simulink subsystem "Guiado2"  (R2021b)
settings: Solver=VariableStepAuto  StartTime=0.0  StopTime=10.0  RelTol=1e-3
values from neighbouring files (symbols this model uses):
  fp = [t1;t2;t3]    [creacionestructurasborrador.m]    (also in flight_plan.m = [sid,wps,iap]; flight_plan_eval.m = [t1;tabla2;t3]; flight_plan_old.m = [sid,wps,iap]; flight_plan_struct.m = [t1;tabla2;t3])
libraries: simulink x5
settings Model: Creator=patri  LastModifiedBy=verti

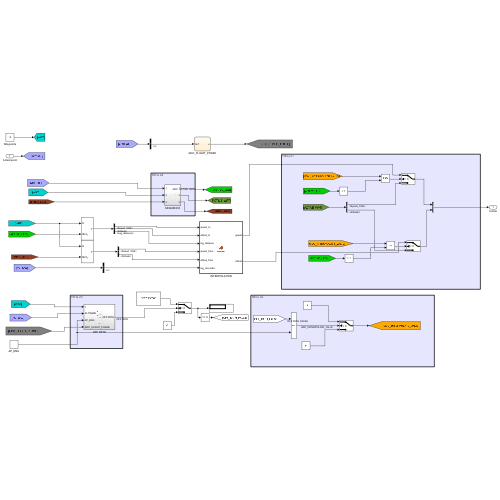
[thumbnail: Simulink's stored preview of the top-level diagram]
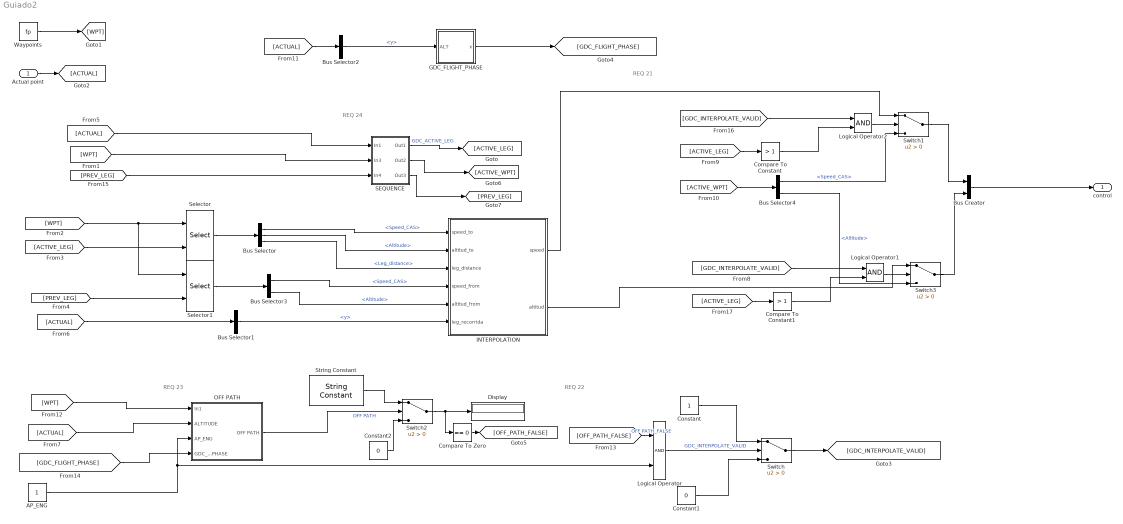
== system Guiado2 ==
  note: REQ 24
  note: REQ 23
  note: REQ 22
  note: REQ 21
  Actual point : Inport  RequirementInfo={} %GIDa_16dc30b3_4c57_4f20_ae6f_49b6e7f70ca9
  AP_ENG : Constant  RequirementInfo={} %GIDa_6cfd0b15_e0b7_412e_b898_13df53d186b9
  Bus Creator : BusCreator  RequirementInfo={} %GIDa_f95eb603_7edc_47e9_9511_efe566d1f221  Inputs=2
  Bus Selector : BusSelector  RequirementInfo={} %GIDa_748c13b4_26a4_4f06_b41f_6c0f351aa6e1  OutputSignals=Speed_CAS,Altitude,Leg_distance
  Bus Selector1 : BusSelector  RequirementInfo={} %GIDa_3209a6ab_bd8c_441c_92f5_266385c658f5  OutputSignals=x; y; z; phi; theta; psi.y
  Bus Selector2 : BusSelector  RequirementInfo={} %GIDa_66241123_1541_4933_9326_b685100fe374  OutputSignals=x; y; z; phi; theta; psi.y
  Bus Selector3 : BusSelector  RequirementInfo={} %GIDa_962e6f27_d2e9_4d95_8ffb_528ca1f04bd7  OutputSignals=Speed_CAS,Altitude
  Bus Selector4 : BusSelector  RequirementInfo={} %GIDa_8319d33c_1374_4958_9d6f_b54157dc937b  OutputSignals=Speed_CAS,Altitude
  Compare To Constant : simulink/Logic and Bit Operations/Compare To Constant  relop=>  const=1  OutDataTypeStr=boolean
  Compare To Constant1 : simulink/Logic and Bit Operations/Compare To Constant  relop=>  const=1  OutDataTypeStr=boolean
  Compare To Zero : simulink/Logic and Bit Operations/Compare To Zero  relop===  OutDataTypeStr=boolean
  Constant : Constant  RequirementInfo={} %GIDa_b37b12f2_4207_4d8d_8f51_6f8b678f3f25
  Constant1 : Constant  RequirementInfo={} %GIDa_9998b814_7f70_4580_aaca_dde72b20b372  Value=0
  Constant2 : Constant  RequirementInfo={} %GIDa_22a48ef9_4669_4f4b_8c84_0df911214b19  Value=0
  Display : Display
      settings: RequirementInfo={} %GIDa_b98bbcc7_d7c3_4a86_b2f1_97de43cdc8ad
  GDC_FLIGHT_PHASE : Stateflow chart  RequirementInfo={} %GIDa_6ca26d66_91a8_4b10_b43c_38c0903f28df  TreatAsAtomicUnit=on
  INTERPOLATION : MATLAB Function  RequirementInfo={} %GIDa_00da5b89_cd18_4ad3_bdd9_46f4b2278232  TreatAsAtomicUnit=on
  Logical Operator : Logic  RequirementInfo={} %GIDa_b237b72d_01a0_4ce8_b8fa_48e4c02eadaf  AllPortsSameDT=off  OutDataTypeStr=boolean
  Logical Operator1 : Logic  RequirementInfo={} %GIDa_3d17652f_edbe_41ba_a049_3408f2c4d262  AllPortsSameDT=off  OutDataTypeStr=boolean
  Logical Operator2 : Logic  RequirementInfo={} %GIDa_1178bee0_2321_439a_8aef_ffe83aa0f831  AllPortsSameDT=off  OutDataTypeStr=boolean
  OFF PATH : Subsystem  RequirementInfo={} %GIDa_e64eeec9_5eff_4758_836b_1b8b16284f0e
  SEQUENCE : Subsystem  RequirementInfo={} %GIDa_19bbec03_9c6d_4828_8024_6321fbffa4bc
  Selector : Selector  RequirementInfo={} %GIDa_52603b66_c8a4_4acb_b10d_5686338dd3d7  InputPortWidth=12  IndexOptions=Index vector (port)  Indices=[1 3]  OutputSizes=1
  Selector1 : Selector  RequirementInfo={} %GIDa_aadcde5b_c971_450e_aee0_b769e6a2f6d5  InputPortWidth=12  IndexOptions=Index vector (port)  Indices=[1 3]  OutputSizes=1
  String Constant : StringConstant  RequirementInfo={} %GIDa_0fff4776_2fb3_4bfd_9582_badec0246361  String="\"OFF PATH\""
  Switch : Switch  RequirementInfo={} %GIDa_7dce933e_33fe_4e3b_ae91_f92ffa975dd8  Criteria=u2 > Threshold
  Switch1 : Switch  RequirementInfo={} %GIDa_97a5f68e_f779_45d0_8fdd_ea3c790676b8  Criteria=u2 > Threshold
  Switch2 : Switch  RequirementInfo={} %GIDa_40c3c411_b3ce_405b_a9d1_145fd5b4c1df  Criteria=u2 > Threshold
  Switch3 : Switch  RequirementInfo={} %GIDa_aa545fae_3300_4656_9f8b_8d88f1b9a628  Criteria=u2 > Threshold
  Waypoints : Constant  RequirementInfo={} %GIDa_99d4dde1_a944_4af8_abed_c7d03318dd1c  Value=fp  OutDataTypeStr=Bus: BUS_FP
  control : Outport  RequirementInfo={} %GIDa_f06892af_3b8f_4cad_820d_58187372560f
  wires:
  SEQUENCE/1(Out1) -> [ACTIVE_LEG]  "GDC_ACTIVE_LEG"
  [PREV_LEG] -> SEQUENCE/3(In4)
  Waypoints/1 -> [WPT]
  [WPT] -> SEQUENCE/2(In3)
  [WPT] -> Selector/1, Selector1/1
  Selector/1 -> Bus Selector/1
  [ACTIVE_LEG] -> Selector/2
  Bus Selector/1 -> INTERPOLATION/1(speed_to)  "<Speed_CAS>"
  Bus Selector/2 -> INTERPOLATION/2(altitud_to)  "<Altitude>"
  Actual point/1 -> [ACTUAL]
  [ACTUAL] -> SEQUENCE/1(In1)
  [ACTUAL] -> Bus Selector1/1
  [ACTUAL] -> OFF PATH/2(ALTITUDE)
  AP_ENG/1 -> Logical Operator/2, OFF PATH/3(AP_ENG)
  OFF PATH/1(OFF PATH) -> Switch2/2  "OFF PATH"
  Logical Operator/1 -> Switch/2  "GDC_INTERPOLATE_VALID"
  Switch/1 -> [GDC_INTERPOLATE_VALID]
  Constant/1 -> Switch/1
  Constant1/1 -> Switch/3
  [GDC_INTERPOLATE_VALID] -> Logical Operator2/1
  [ACTIVE_LEG] -> Compare To Constant/1
  Compare To Constant/1 -> Logical Operator2/2
  Logical Operator2/1 -> Switch1/2
  Bus Selector2/1 -> GDC_FLIGHT_PHASE/1(ALT)  "<y>"
  [ACTUAL] -> Bus Selector2/1
  GDC_FLIGHT_PHASE/1(x) -> [GDC_FLIGHT_PHASE]
  [WPT] -> OFF PATH/1(In1)
  String Constant/1 -> Switch2/1
  Switch2/1 -> Compare To Zero/1, Display/1
  Constant2/1 -> Switch2/3
  [OFF_PATH_FALSE] -> Logical Operator/1  "OFF PATH_FALSE"
  SEQUENCE/2(Out2) -> [ACTIVE_WPT]
  SEQUENCE/3(Out3) -> [PREV_LEG]
  [GDC_FLIGHT_PHASE] -> OFF PATH/4(GDC_FLIGHT_PHASE)
  [PREV_LEG] -> Selector1/2
  Selector1/1 -> Bus Selector3/1
  Bus Selector3/1 -> INTERPOLATION/4(speed_from)  "<Speed_CAS>"
  Bus Selector3/2 -> INTERPOLATION/5(altitud_from)  "<Altitude>"
  INTERPOLATION/1(speed) -> Switch1/1
  [ACTIVE_WPT] -> Bus Selector4/1
  Bus Selector4/1 -> Switch1/3  "<Speed_CAS>"
  INTERPOLATION/2(altitud) -> Switch3/1
  Compare To Constant1/1 -> Logical Operator1/2
  [ACTIVE_LEG] -> Compare To Constant1/1
  [GDC_INTERPOLATE_VALID] -> Logical Operator1/1
  Logical Operator1/1 -> Switch3/2
  Bus Selector4/2 -> Switch3/3  "<Altitude>"
  Bus Creator/1 -> control/1
  Switch1/1 -> Bus Creator/1
  Switch3/1 -> Bus Creator/2
  Bus Selector/3 -> INTERPOLATION/3(leg_distance)  "<Leg_distance>"
  Bus Selector1/1 -> INTERPOLATION/6(leg_recorrida)  "<y>"
  Compare To Zero/1 -> [OFF_PATH_FALSE]

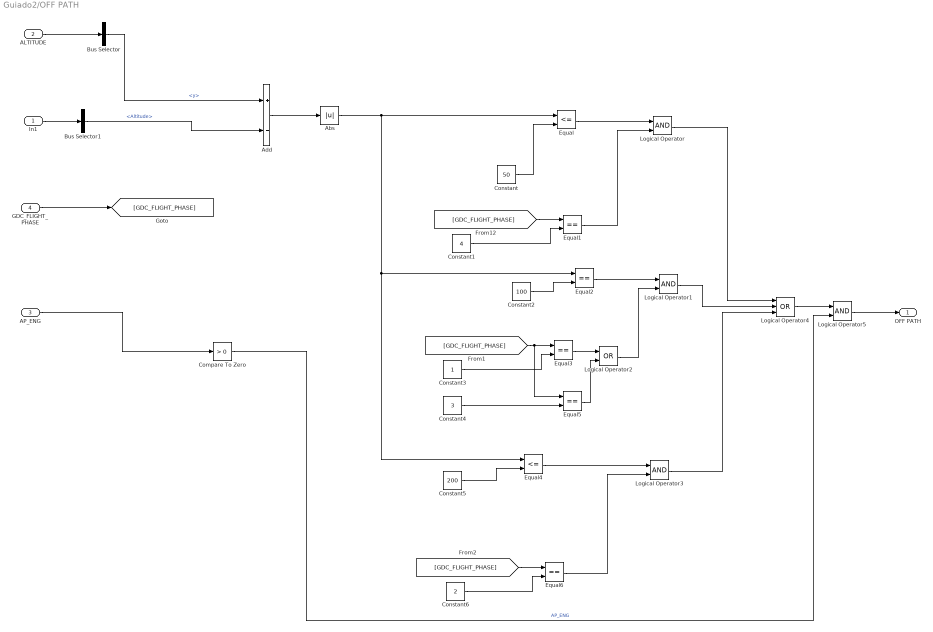
== system Guiado2/OFF PATH ==
  In1 : Inport  RequirementInfo={} %GIDa_62d6845d_2c83_4218_8ed5_ea4377ab5151
  ALTITUDE : Inport  RequirementInfo={} %GIDa_9ea31f00_8010_42f0_928c_ddcfbd884370  Port=2
  AP_ENG : Inport  RequirementInfo={} %GIDa_ee91ff1a_ab3d_4807_8f89_07a74f131ae5  Port=3
  GDC_FLIGHT_PHASE : Inport  RequirementInfo={} %GIDa_dae7e5fb_86bd_4482_b14f_0edc6d3d11c9  Port=4
  Abs : Abs  RequirementInfo={} %GIDa_3a6c06fc_ca93_4cf4_922a_74b5cd0bf12b
  Add : Sum  RequirementInfo={} %GIDa_62393710_84da_4880_81fd_b48a5142b0ab  Inputs=+-
  Bus Selector : BusSelector  RequirementInfo={} %GIDa_3537ae3d_a00e_41d7_b122_9f4ee9b7e234  OutputSignals=x; y; z; phi; theta; psi.y
  Bus Selector1 : BusSelector  RequirementInfo={} %GIDa_83aecc4c_d4cc_4dc5_b0bf_080722190f3a  OutputSignals=Altitude
  Compare To Zero : simulink/Logic and Bit Operations/Compare To Zero  RequirementInfo={} %GIDa_10f91483_6a15_433b_9377_e6e7499d1f49  relop=>  OutDataTypeStr=boolean
  Constant : Constant  RequirementInfo={} %GIDa_9b56d611_43a9_4f81_8a37_8310ab01972c  Value=50
  Constant1 : Constant  RequirementInfo={} %GIDa_6c81b280_bb28_483b_9de7_a5d2e6c184b3  Value=4
  Constant2 : Constant  RequirementInfo={} %GIDa_43ae1b03_ffdd_4284_a340_920d10f39b4e  Value=100
  Constant3 : Constant  RequirementInfo={} %GIDa_2899eea0_8d79_4841_acad_6c949baede0c
  Constant4 : Constant  RequirementInfo={} %GIDa_023f6fee_60f9_4c0a_9384_cd2105696549  Value=3
  Constant5 : Constant  RequirementInfo={} %GIDa_bf05bd0f_ad96_4653_ba6c_864afd652a73  Value=200
  Constant6 : Constant  RequirementInfo={} %GIDa_fbc4b4dc_b940_4f18_bcc6_343711a58847  Value=2
  Equal : RelationalOperator  RequirementInfo={} %GIDa_41fc17ac_0583_4b32_a798_806287f1de59  Operator=<=  OutDataTypeStr=boolean  RndMeth=Simplest
  Equal1 : RelationalOperator  RequirementInfo={} %GIDa_6b358ab3_1c30_4203_b31d_1b7c47e65652  Operator===  OutDataTypeStr=boolean  RndMeth=Simplest
  Equal2 : RelationalOperator  RequirementInfo={} %GIDa_a1929ec3_10c6_4581_ba38_0b3e6f4a191d  Operator===  OutDataTypeStr=boolean  RndMeth=Simplest
  Equal3 : RelationalOperator  RequirementInfo={} %GIDa_ee58c8fd_0997_4c1b_9fda_8de655ddb8c2  Operator===  OutDataTypeStr=boolean  RndMeth=Simplest
  Equal4 : RelationalOperator  RequirementInfo={} %GIDa_40b0daee_de42_4601_9a17_7606db32d086  Operator=<=  OutDataTypeStr=boolean  RndMeth=Simplest
  Equal5 : RelationalOperator  RequirementInfo={} %GIDa_144482dd_7c5e_44de_80d4_0aae76d53f67  Operator===  OutDataTypeStr=boolean  RndMeth=Simplest
  Equal6 : RelationalOperator  RequirementInfo={} %GIDa_2cde3331_25b0_452d_90eb_a86eb0afbb20  Operator===  OutDataTypeStr=boolean  RndMeth=Simplest
  Logical Operator : Logic  RequirementInfo={} %GIDa_948a8364_549f_4376_beca_c4b6c0c4cff5  AllPortsSameDT=off  OutDataTypeStr=boolean
  Logical Operator1 : Logic  RequirementInfo={} %GIDa_cdaccc45_64a9_4082_a1c5_823a8b02242a  AllPortsSameDT=off  OutDataTypeStr=boolean
  Logical Operator2 : Logic  RequirementInfo={} %GIDa_a0c82861_09a2_4c7b_9dd2_c1b7ada60be2  Operator=OR  AllPortsSameDT=off  OutDataTypeStr=boolean
  Logical Operator3 : Logic  RequirementInfo={} %GIDa_b728a0d8_0167_4e3d_a63e_9217ce564790  AllPortsSameDT=off  OutDataTypeStr=boolean
  Logical Operator4 : Logic  RequirementInfo={} %GIDa_947655ff_950d_47b8_be2d_febc351f2bf5  Operator=OR  Inputs=3  AllPortsSameDT=off  OutDataTypeStr=boolean
  Logical Operator5 : Logic  RequirementInfo={} %GIDa_dd42a912_7c92_408c_9973_6a99deedb9ee  AllPortsSameDT=off  OutDataTypeStr=boolean
  OFF PATH : Outport  RequirementInfo={} %GIDa_6c8191e8_8929_43a1_b5d7_c504838d9f7d
  wires:
  GDC_FLIGHT_PHASE/1 -> [GDC_FLIGHT_PHASE]
  Logical Operator5/1 -> OFF PATH/1
  Bus Selector1/1 -> Add/2  "<Altitude>"
  Logical Operator4/1 -> Logical Operator5/1
  Logical Operator3/1 -> Logical Operator4/3
  Logical Operator1/1 -> Logical Operator4/2
  Logical Operator/1 -> Logical Operator4/1
  Equal4/1 -> Logical Operator3/1
  Equal6/1 -> Logical Operator3/2
  [GDC_FLIGHT_PHASE] -> Equal6/1
  Constant6/1 -> Equal6/2
  Constant5/1 -> Equal4/2
  Logical Operator2/1 -> Logical Operator1/2
  Equal5/1 -> Logical Operator2/2
  Constant4/1 -> Equal5/2
  Equal3/1 -> Logical Operator2/1
  Equal2/1 -> Logical Operator1/1
  [GDC_FLIGHT_PHASE] -> Equal3/1, Equal5/1
  Constant3/1 -> Equal3/2
  Constant2/1 -> Equal2/2
  Equal/1 -> Logical Operator/1
  Equal1/1 -> Logical Operator/2
  Constant1/1 -> Equal1/2
  [GDC_FLIGHT_PHASE] -> Equal1/1
  Abs/1 -> Equal/1, Equal2/1, Equal4/1
  Constant/1 -> Equal/2
  Add/1 -> Abs/1
  Bus Selector/1 -> Add/1  "<y>"
  In1/1 -> Bus Selector1/1
  ALTITUDE/1 -> Bus Selector/1
  Compare To Zero/1 -> Logical Operator5/2  "AP_ENG"
  AP_ENG/1 -> Compare To Zero/1

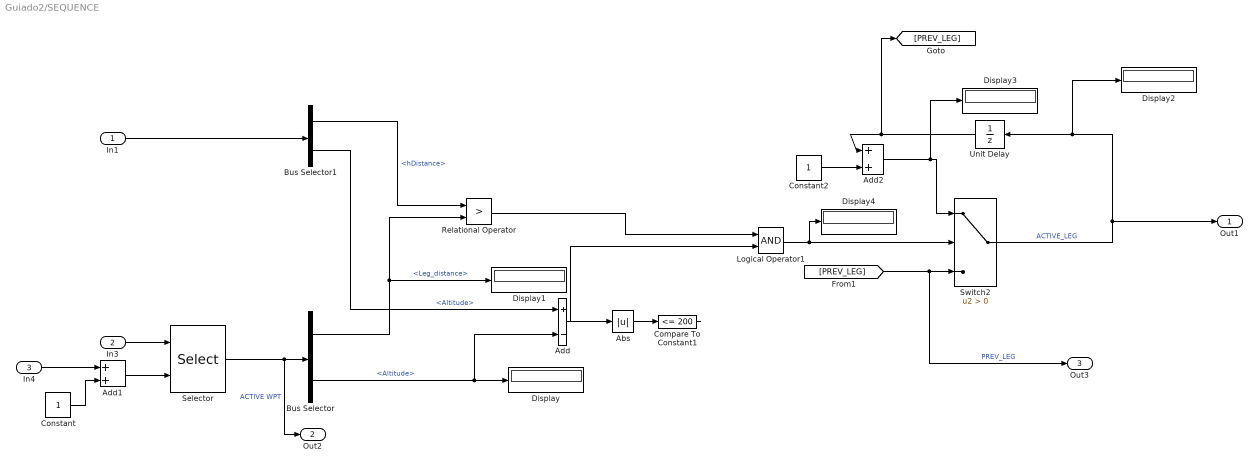
== system Guiado2/SEQUENCE ==
  In1 : Inport
  In3 : Inport  Port=2
  In4 : Inport  Port=3
  Abs : Abs
  Add : Sum  Inputs=+-
  Add1 : Sum
  Add2 : Sum
  Bus Selector : BusSelector  OutputSignals=Leg_distance,Altitude
  Bus Selector1 : BusSelector  OutputSignals=hDistance,Altitude
  Compare To Constant1 : simulink/Logic and Bit Operations/Compare To Constant  relop=<=  const=200  OutDataTypeStr=boolean
  Constant : Constant
  Constant2 : Constant
  Display{,1..4} (5 alike) : Display
  Logical Operator1 : Logic  AllPortsSameDT=off  OutDataTypeStr=boolean
  Relational Operator : RelationalOperator  Operator=>  OutDataTypeStr=boolean  RndMeth=Simplest
  Selector : Selector  InputPortWidth=12  IndexOptions=Index vector (port)  Indices=[1 3]  OutputSizes=1
  Switch2 : Switch  Criteria=u2 > Threshold
  Unit Delay : UnitDelay  SampleTime=-1  HasFrameUpgradeWarning=on
  Out1 : Outport
  Out2 : Outport  Port=2
  Out3 : Outport  Port=3
  wires:
  Constant2/1 -> Add2/2
  Bus Selector/2 -> Add/2, Display/1  "<Altitude>"
  Logical Operator1/1 -> Display4/1, Switch2/2
  Switch2/1 -> Out1/1, Display2/1, Unit Delay/1  "ACTIVE_LEG"
  Bus Selector1/1 -> Relational Operator/1  "<hDistance>"
  Abs/1 -> Compare To Constant1/1
  In4/1 -> Add1/1
  Unit Delay/1 -> Add2/1, [PREV_LEG]
  Bus Selector/1 -> Display1/1, Relational Operator/2  "<Leg_distance>"
  Relational Operator/1 -> Logical Operator1/1
  Bus Selector1/2 -> Add/1  "<Altitude>"
  In1/1 -> Bus Selector1/1
  Compare To Constant1/1 -> Logical Operator1/2
  Add2/1 -> Display3/1, Switch2/1
  Add/1 -> Abs/1
  In3/1 -> Selector/1
  Selector/1 -> Out2/1, Bus Selector/1  "ACTIVE WPT"
  Constant/1 -> Add1/2
  [PREV_LEG] -> Switch2/3, Out3/1  "PREV_LEG"
  Add1/1 -> Selector/2

== matlab function Guiado2/INTERPOLATION ==
  data: speed_to input; altitud_to input; leg_distance input; speed_from input; altitud_from input; leg_recorrida input; speed output; altitud output
function [speed,altitud] = mapeo(speed_to,altitud_to,leg_distance,speed_from,altitud_from,leg_recorrida)

speed = (leg_recorrida) .* (speed_to - speed_from) ./ (leg_distance) + speed_from;
altitud = (leg_recorrida) .* (altitud_to - altitud_from) ./ (leg_distance) + altitud_from;

end

== stateflow chart Guiado2/GDC_FLIGHT_PHASE ==
  state CLIMB
    entry:
    x==1;
  state CRUISE
    entry:
    x==2;
  state DESCEND
    entry:
    x==3;
  state APPROACH
    entry:
    x==4;
  (default) -> CLIMB
  DESCEND -> APPROACH : [ALT<2000]
  CLIMB -> CRUISE : [ALT>=CRZ_ALT]
  CRUISE -> DESCEND [order 2] : [(ALT<CRZ_ALT) & (ENG_RAT==IDLE)]
  CRUISE -> CLIMB [order 1] : [ALT<CRZ_ALT & (ENG_RAT==MTO | ENG_RAT==MCT | ENG_RAT==CLB)]
  data: ALT input; x output; CRZ_ALT local; CLB local; MTO local
